simulink model "deltino"  (R2021b)
settings: Solver=VariableStepAuto  StartTime=0.0  StopTime=inf  FixedStep=0.0001  RelTol=1e-3
values from neighbouring files (symbols this model uses):
  alpha1 = 0    [compute_deltino_dyn_parallel.m]
  alpha2 = 2/3*pi    (= 2.09439510239)    [compute_deltino_dyn_parallel.m]
  alpha3 = 4/3*pi    (= 4.18879020479)    [compute_deltino_dyn_parallel.m]
  H = 0.05    [main.m]
  J_T = [J_1', J_2', J_3', J_4']    [main.m]
  K_d = 10    [main.m]
  K_el = 10000    [main.m]
  K_i = 1    [main.m]
  K_p = 200    [main.m]
  K_v = 10    [main.m]
  mu = 0.8    [main.m]
  ni_0 = zeros(18,1)    [main.m]
  offset1 = [l1/2; l2/2; -h/2]    [compute_deltino_dyn_parallel.m]    (also in main.m = [+l1/2; +l2/2; -h/2])
  offset2 = [l1/2; -l2/2; -h/2]    [compute_deltino_dyn_parallel.m]    (also in main.m = [+l1/2; -l2/2; -h/2])
  offset3 = [-l1/2; -l2/2; -h/2]    [compute_deltino_dyn_parallel.m]    (also in main.m)
  offset4 = [-l1/2; l2/2; -h/2]    [compute_deltino_dyn_parallel.m]    (also in main.m = [-l1/2; +l2/2; -h/2])
  p_leg1_0 = forward_kin(theta_leg1_0)    [main.m]
  p_leg2_0 = forward_kin(theta_leg2_0)    [main.m]
  p_leg3_0 = forward_kin(theta_leg3_0)    [main.m]
  p_leg4_0 = forward_kin(theta_leg4_0)    [main.m]
  points_ccw = [+0.1,  0.00 ... (first row only)    [main.m]
  points_cw = [-0.1,  0.00 ... (first row only)    [main.m]
  q_0 = [base_0; ypr_0; theta_leg1_0; ee_leg1_0; theta_leg2_0; ee_leg2_0;        theta_leg3_0; ee_leg3_0; theta_leg4_0; ee_leg4_0;]    [main.m]
  ratio = 2    [main.m]
  steps = 4+2*ratio    (= 8)    [main.m]
  theta_leg1_0 = [pi/6; pi/6; pi/6]    [main.m]
  theta_leg2_0 = [pi/6; pi/6; pi/6]    [main.m]
  theta_leg3_0 = [pi/6; pi/6; pi/6]    [main.m]
  theta_leg4_0 = [pi/6; pi/6; pi/6]    [main.m]
  ts = T/steps    (= 0.1875)    [main.m]
  ts2 = 3*ts    (= 0.5625)    [main.m]
  vel = 0.2    [main.m]
undefined symbols (not defined in the file or in its folder): l1, l_A, l_B, R, radius0, radius1, radius2, theta, WPs
libraries: simulink x14, dspsigops x12
(part 5 of 10)

== matlab function deltino/TRAJ PLANNING/legs traj generator rotate/leg_generator1/MATLAB Function ==
  data: u1 input; y output; u2 input
function y = OR(u1, u2)

if (u1==0) && (u2==0)
    y = 0;
else 
    y = 1;
end

== matlab function deltino/TRAJ PLANNING/legs traj generator rotate/leg_generator1/swing rotate ==
  data: t input; alpha input; pos output; H parameter; ts2 parameter; l1 parameter; offset1 parameter

function pos = fcn(t, alpha, H, ts2, l1, offset1)

T_BD1 = R_z(-(pi+pi/2+pi/4+alpha))*T_x(sqrt(2)*l1/2);
d_B = T_BD1(1:3,4);
d_B1 = d_B - offset1;

x_0 = 0;
x_1 = d_B1(1) ;
    x1 = x_0;
    x2 = 0;
    x3 = 0;
    x4 = (10*(x_1 - x_0))/ts2^3;
    x5 = -(15*(x_1 - x_0))/ts2^4;
    x6 = (6*(x_1 - x_0))/ts2^5;
x = x1 + x2*t + x3*t^2 + x4*t^3 +x5*t^4 + x6*t^5;

y_0 = 0;
y_1 = d_B1(2);
    y1 = y_0;
    y2 = 0;
    y3 = 0;
    y4 = (10*(y_1 - y_0))/ts2^3;
    y5 = -(15*(y_1 - y_0))/ts2^4;
    y6 = (6*(y_1 - y_0))/ts2^5;
y = y1 + y2*t + y3*t^2 + y4*t^3 + y5*t^4 + y6*t^5;

z = H/2*(1 - cos(2*pi*t/ts2));

pos = [x;y;z];

== matlab function deltino/TRAJ PLANNING/legs traj generator rotate/leg_generator2/MATLAB Function ==
  data: u1 input; y output; u2 input
function y = OR(u1, u2)

if (u1==0) && (u2==0)
    y = 0;
else 
    y = 1;
end

== matlab function deltino/TRAJ PLANNING/legs traj generator rotate/leg_generator2/swing rotate ==
  data: t input; alpha input; pos output; H parameter; ts2 parameter; l1 parameter; offset2 parameter

function pos = fcn(t, alpha, H, ts2, l1, offset2)

T_BD2 = R_z(-(pi/4+alpha))*T_x(sqrt(2)*l1/2);
d_B = T_BD2(1:3,4);
d_B2 = d_B - offset2;

x_0 = 0;
x_1 = d_B2(1) ;
    x1 = x_0;
    x2 = 0;
    x3 = 0;
    x4 = (10*(x_1 - x_0))/ts2^3;
    x5 = -(15*(x_1 - x_0))/ts2^4;
    x6 = (6*(x_1 - x_0))/ts2^5;
x = x1 + x2*t + x3*t^2 + x4*t^3 +x5*t^4 + x6*t^5;

y_0 = 0;
y_1 = d_B2(2);
    y1 = y_0;
    y2 = 0;
    y3 = 0;
    y4 = (10*(y_1 - y_0))/ts2^3;
    y5 = -(15*(y_1 - y_0))/ts2^4;
    y6 = (6*(y_1 - y_0))/ts2^5;
y = y1 + y2*t + y3*t^2 + y4*t^3 + y5*t^4 + y6*t^5;

z = H/2*(1 - cos(2*pi*t/ts2));

pos = [x;y;z];

== matlab function deltino/TRAJ PLANNING/ Encoder ==
  data: u1 input; ctrl input; u2 input; y1 output; y2 output; y3 output; y4 output; p_leg2_0 parameter; p_leg1_0 parameter; p_leg3_0 parameter; p_leg4_0 parameter
function [y1, y2, y3, y4] = encoder(u1, ctrl, u2, p_leg2_0, p_leg1_0, p_leg3_0, p_leg4_0)
    y1 = p_leg1_0;
    y2 = p_leg2_0;
    y3 = p_leg3_0;
    y4 = p_leg4_0;
    
    if ctrl == 1 % forth
        y1 = Rz(0)*u1(1:3);
        y2 = Rz(0)*u1(4:6);
        y3 = Rz(0)*u1(7:9);
        y4 = Rz(0)*u1(10:12);
    elseif ctrl == 3 % back
        y1 = Rz(pi)*u1(1:3);
        y2 = Rz(pi)*u1(4:6);
        y3 = Rz(pi)*u1(7:9);
        y4 = Rz(pi)*u1(10:12);
    elseif ctrl == 2 % right
        y1 = Rz(-pi/2)*u1(1:3);
        y2 = Rz(-pi/2)*u1(4:6);
        y3 = Rz(-pi/2)*u1(7:9);
        y4 = Rz(-pi/2)*u1(10:12);
	elseif ctrl == 4 % left
        y1 = Rz(pi/2)*u1(1:3);
        y2 = Rz(pi/2)*u1(4:6);
        y3 = Rz(pi/2)*u1(7:9);
        y4 = Rz(pi/2)*u1(10:12);
    elseif (ctrl == 5) || (ctrl==6)
        y1 = u2(1:3);
        y2 = u2(4:6);
        y3 = u2(7:9);
        y4 = u2(10:12);
    end

== matlab function deltino/TRAJ PLANNING/MATLAB Function ==
  data: mode input; alpha input; real_alpha output
function real_alpha = fcn(mode, alpha)

if mode == 5
    real_alpha = alpha;
else 
    real_alpha = -alpha;
end

== matlab function deltino/TRAJ PLANNING/legs traj generator rotate/leg_generator3/MATLAB Function ==
  data: u1 input; y output; u2 input
function y = OR(u1, u2)

if (u1==0) && (u2==0)
    y = 0;
else 
    y = 1;
end

== matlab function deltino/TRAJ PLANNING/legs traj generator rotate/leg_generator3/swing rotate ==
  data: t input; alpha input; pos output; H parameter; ts2 parameter; l1 parameter; offset3 parameter

function pos = fcn(t, alpha, H, ts2, l1, offset3)

T_BD3 = R_z(-(pi/2+pi/4+alpha))*T_x(sqrt(2)*l1/2);
d_B = T_BD3(1:3,4);
d_B3 = d_B - offset3;

x_0 = 0;
x_1 = d_B3(1) ;
    x1 = x_0;
    x2 = 0;
    x3 = 0;
    x4 = (10*(x_1 - x_0))/ts2^3;
    x5 = -(15*(x_1 - x_0))/ts2^4;
    x6 = (6*(x_1 - x_0))/ts2^5;
x = x1 + x2*t + x3*t^2 + x4*t^3 +x5*t^4 + x6*t^5;

y_0 = 0;
y_1 = d_B3(2);
    y1 = y_0;
    y2 = 0;
    y3 = 0;
    y4 = (10*(y_1 - y_0))/ts2^3;
    y5 = -(15*(y_1 - y_0))/ts2^4;
    y6 = (6*(y_1 - y_0))/ts2^5;
y = y1 + y2*t + y3*t^2 + y4*t^3 + y5*t^4 + y6*t^5;

z = H/2*(1 - cos(2*pi*t/ts2));

pos = [x;y;z];

== matlab function deltino/TRAJ PLANNING/legs traj generator rotate/leg_generator4/MATLAB Function ==
  data: u1 input; y output; u2 input
function y = OR(u1, u2)

if (u1==0) && (u2==0)
    y = 0;
else 
    y = 1;
end

== matlab function deltino/TRAJ PLANNING/legs traj generator rotate/leg_generator4/swing rotate ==
  data: t input; alpha input; pos output; H parameter; ts2 parameter; l1 parameter; offset4 parameter

function pos = fcn(t, alpha, H, ts2, l1, offset4)

T_BD4 = R_z(-(pi+pi/4+alpha))*T_x(sqrt(2)*l1/2);
d_B = T_BD4(1:3,4);
d_B4 = d_B - offset4;

x_0 = 0;
x_1 = d_B4(1) ;
    x1 = x_0;
    x2 = 0;
    x3 = 0;
    x4 = (10*(x_1 - x_0))/ts2^3;
    x5 = -(15*(x_1 - x_0))/ts2^4;
    x6 = (6*(x_1 - x_0))/ts2^5;
x = x1 + x2*t + x3*t^2 + x4*t^3 +x5*t^4 + x6*t^5;

y_0 = 0;
y_1 = d_B4(2);
    y1 = y_0;
    y2 = 0;
    y3 = 0;
    y4 = (10*(y_1 - y_0))/ts2^3;
    y5 = -(15*(y_1 - y_0))/ts2^4;
    y6 = (6*(y_1 - y_0))/ts2^5;
y = y1 + y2*t + y3*t^2 + y4*t^3 + y5*t^4 + y6*t^5;

z = H/2*(1 - cos(2*pi*t/ts2));

pos = [x;y;z];

== matlab function deltino/TRAJ PLANNING/legs traj generator rotate/leg_generator1/swing rotate back ==
  data: t input; alpha input; pos output; ts2 parameter; l1 parameter; offset1 parameter

function pos = fcn(t, alpha, ts2, l1, offset1)

T_BD1 = R_z(-(pi+pi/2+pi/4+alpha))*T_x(sqrt(2)*l1/2);
d_B = T_BD1(1:3,4);
d_B1 = d_B - offset1;

x_0 = d_B1(1);
x_1 = 0;
    x1 = x_0;
    x2 = 0;
    x3 = 0;
    x4 = (10*(x_1 - x_0))/ts2^3;
    x5 = -(15*(x_1 - x_0))/ts2^4;
    x6 = (6*(x_1 - x_0))/ts2^5;
x = x1 + x2*t + x3*t^2 + x4*t^3 +x5*t^4 + x6*t^5;

y_0 = d_B1(2);
y_1 = 0;
    y1 = y_0;
    y2 = 0;
    y3 = 0;
    y4 = (10*(y_1 - y_0))/ts2^3;
    y5 = -(15*(y_1 - y_0))/ts2^4;
    y6 = (6*(y_1 - y_0))/ts2^5;
y = y1 + y2*t + y3*t^2 + y4*t^3 + y5*t^4 + y6*t^5;

pos = [x;y;0];

== matlab function deltino/TRAJ PLANNING/legs traj generator rotate/leg_generator2/swing rotate back ==
  data: t input; alpha input; pos output; ts2 parameter; l1 parameter; offset2 parameter

function pos = fcn(t, alpha, ts2, l1, offset2)

T_BD2 = R_z(-(pi/4+alpha))*T_x(sqrt(2)*l1/2);
d_B = T_BD2(1:3,4);
d_B2 = d_B - offset2;

x_0 = d_B2(1);
x_1 = 0;
    x1 = x_0;
    x2 = 0;
    x3 = 0;
    x4 = (10*(x_1 - x_0))/ts2^3;
    x5 = -(15*(x_1 - x_0))/ts2^4;
    x6 = (6*(x_1 - x_0))/ts2^5;
x = x1 + x2*t + x3*t^2 + x4*t^3 +x5*t^4 + x6*t^5;

y_0 = d_B2(2);
y_1 = 0;
    y1 = y_0;
    y2 = 0;
    y3 = 0;
    y4 = (10*(y_1 - y_0))/ts2^3;
    y5 = -(15*(y_1 - y_0))/ts2^4;
    y6 = (6*(y_1 - y_0))/ts2^5;
y = y1 + y2*t + y3*t^2 + y4*t^3 + y5*t^4 + y6*t^5;

pos = [x;y;0];

== matlab function deltino/TRAJ PLANNING/legs traj generator rotate/leg_generator3/swing rotate back ==
  data: t input; alpha input; pos output; ts2 parameter; l1 parameter; offset3 parameter

function pos = fcn(t, alpha, ts2, l1, offset3)

T_BD3 = R_z(-(pi/2+pi/4+alpha))*T_x(sqrt(2)*l1/2);
d_B = T_BD3(1:3,4);
d_B3 = d_B - offset3;

x_0 = d_B3(1);
x_1 = 0;
    x1 = x_0;
    x2 = 0;
    x3 = 0;
    x4 = (10*(x_1 - x_0))/ts2^3;
    x5 = -(15*(x_1 - x_0))/ts2^4;
    x6 = (6*(x_1 - x_0))/ts2^5;
x = x1 + x2*t + x3*t^2 + x4*t^3 +x5*t^4 + x6*t^5;

y_0 = d_B3(2);
y_1 = 0;
    y1 = y_0;
    y2 = 0;
    y3 = 0;
    y4 = (10*(y_1 - y_0))/ts2^3;
    y5 = -(15*(y_1 - y_0))/ts2^4;
    y6 = (6*(y_1 - y_0))/ts2^5;
y = y1 + y2*t + y3*t^2 + y4*t^3 + y5*t^4 + y6*t^5;

pos = [x;y;0];

== matlab function deltino/TRAJ PLANNING/legs traj generator rotate/leg_generator4/swing rotate back ==
  data: t input; alpha input; pos output; ts2 parameter; l1 parameter; offset4 parameter

function pos = fcn(t, alpha, ts2, l1, offset4)

T_BD4 = R_z(-(pi+pi/4+alpha))*T_x(sqrt(2)*l1/2);
d_B = T_BD4(1:3,4);
d_B4 = d_B - offset4;

x_0 = d_B4(1);
x_1 = 0;
    x1 = x_0;
    x2 = 0;
    x3 = 0;
    x4 = (10*(x_1 - x_0))/ts2^3;
    x5 = -(15*(x_1 - x_0))/ts2^4;
    x6 = (6*(x_1 - x_0))/ts2^5;
x = x1 + x2*t + x3*t^2 + x4*t^3 +x5*t^4 + x6*t^5;

y_0 = d_B4(2);
y_1 = 0;
    y1 = y_0;
    y2 = 0;
    y3 = 0;
    y4 = (10*(y_1 - y_0))/ts2^3;
    y5 = -(15*(y_1 - y_0))/ts2^4;
    y6 = (6*(y_1 - y_0))/ts2^5;
y = y1 + y2*t + y3*t^2 + y4*t^3 + y5*t^4 + y6*t^5;

pos = [x;y;0];

== matlab function deltino/WAYPOINTS GENERATOR/MATLAB Function ==
  data: all_WPs input; old_reached input; current_WP output size=[1,2]; reached input; old_last input; new_last output size=1
function [current_WP, new_last]  = fcn(all_WPs, old_reached, reached, old_last)

dim = size(all_WPs);

if old_last < dim(1)
	if reached == 1 && old_reached == 0
		new_last = old_last + 1;
		current_WP = all_WPs(new_last,:);
	else
		new_last = old_last;
		current_WP = all_WPs(new_last,:);
	end
else
	current_WP = all_WPs(old_last,:);
	new_last = old_last;
end

== matlab function deltino/TRAJ PLANNING/legs traj generator rotate/rotate_CW ==
  data: shift output; leg input; t input; points_cw parameter; ts2 parameter
function shift = shift_CoM(leg, t, points_cw, ts2)

X1 = points_cw(1,1);
Y1 = points_cw(1,2);
X2 = points_cw(2,1);
Y2 = points_cw(2,2);
X3 = points_cw(3,1);
Y3 = points_cw(3,2);


shift = [0;0;0];

switch leg
	case 0.5 
		x_0 = 0;
		x_1 = X1;
		x1 = x_0;
		x2 = 0;
		x3 = 0;
		x4 = (10*(x_1 - x_0))/ts2^3;
		x5 = -(15*(x_1 - x_0))/ts2^4;
		x6 = (6*(x_1 - x_0))/ts2^5;
		shiftx = x1 + x2*t + x3*t^2 + x4*t^3 +x5*t^4 + x6*t^5;
	
		y_0 = 0;
		y_1 = Y1;
		y1 = y_0;
		y2 = 0;
		y3 = 0;
		y4 = (10*(y_1 - y_0))/ts2^3;
		y5 = -(15*(y_1 - y_0))/ts2^4;
		y6 = (6*(y_1 - y_0))/ts2^5;
		shifty = y1 + y2*t + y3*t^2 + y4*t^3 + y5*t^4 + y6*t^5;

		shift = [shiftx; shifty; 0];
	case 1 
		shift = [X1; Y1; 0];
	case 2 
		shift = [X1; Y1; 0];
	case 2.5
		x_0 = X1;
		x_1 = X2;
		x1 = x_0;
		x2 = 0;
		x3 = 0;
		x4 = (10*(x_1 - x_0))/ts2^3;
		x5 = -(15*(x_1 - x_0))/ts2^4;
		x6 = (6*(x_1 - x_0))/ts2^5;
		shiftx = x1 + x2*(t-3*ts2) + x3*(t-3*ts2)^2 + x4*(t-3*ts2)^3 +x5*(t-3*ts2)^4 + x6*(t-3*ts2)^5;
	
		y_0 = Y1;
		y_1 = Y2;
		y1 = y_0;
		y2 = 0;
		y3 = 0;
		y4 = (10*(y_1 - y_0))/ts2^3;
		y5 = -(15*(y_1 - y_0))/ts2^4;
		y6 = (6*(y_1 - y_0))/ts2^5;
		shifty = y1 + y2*(t-3*ts2) + y3*(t-3*ts2)^2 + y4*(t-3*ts2)^3 + y5*(t-3*ts2)^4 + y6*(t-3*ts2)^5;
		shift = [shiftx; shifty; 0];
	case 3
		shift = [X2; Y2; 0];
	case 4 
		shift = [X2; Y2; 0];
	case 5
		x_0 = X2;
		x_1 = X3;
		x1 = x_0;
		x2 = 0;
		x3 = 0;
		x4 = (10*(x_1 - x_0))/ts2^3;
		x5 = -(15*(x_1 - x_0))/ts2^4;
		x6 = (6*(x_1 - x_0))/ts2^5;
		shiftx = x1 + x2*(t-6*ts2) + x3*(t-6*ts2)^2 + x4*(t-6*ts2)^3 +x5*(t-6*ts2)^4 + x6*(t-6*ts2)^5;
	
		y_0 = Y2;
		y_1 = Y3;
		y1 = y_0;
		y2 = 0;
		y3 = 0;
		y4 = (10*(y_1 - y_0))/ts2^3;
		y5 = -(15*(y_1 - y_0))/ts2^4;
		y6 = (6*(y_1 - y_0))/ts2^5;
		shifty = y1 + y2*(t-6*ts2) + y3*(t-6*ts2)^2 + y4*(t-6*ts2)^3 + y5*(t-6*ts2)^4 + y6*(t-6*ts2)^5;
		shift = [shiftx; shifty; 0];
end

% 
% switch leg
% 	case 0.5 
% 		shiftx = X1 * t/ts2;
% 		shifty = Y1 * t/ts2;
% 		shift = [shiftx; shifty; 0];
% 	case 1 
% 		shift = [X1; Y1; 0];
% 	case 2 
% 		shift = [X1; Y1; 0];
% 	case 2.5
% 		shiftx = X2 * (t-3*ts2)/ts2 + X1 * (1-(t-3*ts2)/ts2);
% 		shifty = Y2 * (t-3*ts2)/ts2 + Y1 * (1-(t-3*ts2)/ts2);
% 		shift = [shiftx; shifty; 0];
% 	case 3
% 		shift = [X2; Y2; 0];
% 	case 4 
% 		shift = [X2; Y2; 0];
% 	case 5
% 		shiftx = X3 * (t-6*ts2)/ts2 + X2 * (1-(t-6*ts2)/ts2);
% 		shifty = Y3 * (t-6*ts2)/ts2 + Y2 * (1-(t-6*ts2)/ts2);
% 		shift = [shiftx; shifty; 0];
% end

== matlab function deltino/INVERVSE KINEMATICS/Pos_to_Theta ==
  data: pos_Bi input; alpha1 parameter; alpha2 parameter; alpha3 parameter; R parameter; l_A parameter; l_B parameter; theta output; theta_old output; theta_old input
function [theta, theta_old] = inverse_kin(pos_Bi, alpha1, alpha2, alpha3, R, l_A, l_B, theta_old)

    theta = zeros(12,1);

    for idx = 1:4

        % Foot coordinates in frame {B_i}
        p = pos_Bi(1+(idx-1)*3:idx*3);

        % Equations of trilateration to be solved
        F = @(th) [norm(p - Rz(alpha1) * [R+l_A*cos(th(1)); 0; -l_A*sin(th(1))])^2 - l_B^2;
                   norm(p - Rz(alpha2) * [R+l_A*cos(th(2)); 0; -l_A*sin(th(2))])^2 - l_B^2;
                   norm(p - Rz(alpha3) * [R+l_A*cos(th(3)); 0; -l_A*sin(th(3))])^2 - l_B^2];
        x0 = theta_old(1+(idx-1)*3:idx*3);
        opt = optimoptions('fsolve', 'Algorithm', 'levenberg-marquardt');

        [res, val] = fsolve(F, x0, opt);
        theta(1+(idx-1)*3:idx*3) = res;
    end 
    
    theta_old  = theta;
end

== matlab function deltino/CONTACT FORCES/Contact Forces Leg1/Contact Forces ==
  data: p_ee input; f output; v_ee input; contact input; p0 input; contact output; p0 output; K_el parameter; K_v parameter; mu parameter
function [f, contact, p0] = compute_contact_forces(p_ee, v_ee, contact, p0, K_el, K_v, mu)
    f = zeros(3,1);

    if(p_ee(3) < 0)

        % Normal Force
        f_e = -K_el * p_ee(3);
        if(v_ee(3) < 0)
            f_v = f_e * K_v * (-v_ee(3));
        else
            f_v = 0;
        end
        f(3) = f_e + f_v;

        % Tangential Force
        if(contact == 0) % we must initialize x0
            contact = 1;
            p0 = p_ee(1:2);
            f(1:2) = K_el * (p0 - p_ee(1:2)); % == 0 !! 
        else 
            % tangential force computation
            f(1:2) = K_el * (p0 - p_ee(1:2));

            % update of p0_x  
            if(f(1) > mu * f(3))
                p0(1) = (mu * f(3))/K_el + p_ee(1);
                f(1) = mu * f(3);
            elseif(-f(1) > mu * f(3))
                p0(1) = -(mu * f(3))/K_el + p_ee(1);
                f(1) = - mu * f(3);
            end
            
            % update of p0_y
            if(f(2) > mu * f(3))
                p0(2) = (mu * f(3))/K_el + p_ee(2);
                f(2) = mu * f(3);
            elseif(-f(2) > mu * f(3))
                p0(2) = -(mu * f(3))/K_el + p_ee(2);
              f(2) = -mu * f(3);
            end    
        end
     
    else % reset of contact tracking
        contact = 0;
    end

    %f(1) = 0;
    %f(2) = 0;


end

== matlab function deltino/MATLAB Function1 ==
  data: q input; theta output
function theta = select_theta(q)

theta = [q(7:9); q(13:15); q(19:21); q(25:27)];

end

== matlab function deltino/GUIDANCE SYSTEM/MATLAB Function ==
  data: reached output; mode output; velocity output; wp input; alpha output; q input; doing input; radius0 parameter; vel parameter; old_vel input; old_alpha input; radius1 parameter; radius2 parameter; theta parameter
function [reached, mode, velocity, alpha] = ...
	fcn(wp, q, doing, radius0, vel, old_vel, old_alpha, radius1, radius2, theta)

mode = 0;
alpha = old_alpha;
velocity = old_vel; 
reached = 0;

% DO SOMETHING ONLY IF PREVIOUS ACTION IS FINISHED
if doing == 0 

% 1) Check whether WP is reached
x = wp(1) - q(1);
y = wp(2) - q(2);
dist = sqrt(x^2+y^2);
if dist < radius0 
	reached = 1;
else
	theta = theta/180*pi;

	vel1 = vel/2;
	vel2 = vel/4;
	
	% 2) Check for heading
	robot_yaw = q(4);
	heading_des_spatial = atan2(y,x);
	heading_des_robot = heading_des_spatial-robot_yaw;
	heading_des = wrapToPi(heading_des_robot);
	if (-pi/4 < heading_des) && (heading_des <= pi/4)
    	head = 1; % front
    	heading_des = heading_des+0;
	elseif  (pi/4 < heading_des) && (heading_des <= 3/4*pi)
    	head = 4; % left
    	heading_des = heading_des-pi/2;
	elseif (3/4*pi < heading_des)
    	head = 3; % back
    	heading_des = heading_des-pi;
	elseif (heading_des <= -3/4*pi)
    	head = 3; % back
    	heading_des = heading_des+pi; 
	elseif (-3/4*pi < heading_des) && (heading_des <= -pi/4)
    	head = 2; % right
    	heading_des = heading_des+pi/2;
    else
        head = 9;
	end
	
    miss_distance = abs(dist*sin(heading_des));
    angle_error = abs(heading_des);
	if (angle_error > theta) && (miss_distance > radius0)
		adjust = 1;
	else
		adjust = 0;
	end

	if adjust == 0
    	% 3.1) Adjust velocity
    	mode = head;
		if dist < radius2 
        	velocity = vel2;
    	elseif dist < radius1
        	velocity = vel1;
    	else 
        	velocity = vel;
		end
	else
    	% 3.2) Adjust heading
		if heading_des > 0 % rotate counterclockwise
			if abs(heading_des) <= pi/8 % do just one rotation
				mode = 6;
				alpha = abs(heading_des);
			else %do two rotations
				mode = 6;
				alpha = abs(heading_des)/2;
			end
		else % rotate clockwise
			if abs(heading_des) <= pi/8 % do just one rotation
				mode = 5;
				alpha = abs(heading_des);
			else %do two rotations
				mode = 5;
				alpha = abs(heading_des)/2;
			end
		end
		alpha = alpha + 0.1*alpha;
	end

end

end

== matlab function deltino/TRAJ PLANNING/legs traj generator rotate/rotate CCW ==
  data: shift output; leg input; t input; points_ccw parameter; ts2 parameter
function shift  = shift_CoM(leg, t, points_ccw, ts2)

X1 = points_ccw(1,1);
Y1 = points_ccw(1,2);
X2 = points_ccw(2,1);
Y2 = points_ccw(2,2);
X3 = points_ccw(3,1);
Y3 = points_ccw(3,2);

shift = [0;0;0];

switch leg
	case 4.5 
		x_0 = 0;
		x_1 = X1;
		x1 = x_0;
		x2 = 0;
		x3 = 0;
		x4 = (10*(x_1 - x_0))/ts2^3;
		x5 = -(15*(x_1 - x_0))/ts2^4;
		x6 = (6*(x_1 - x_0))/ts2^5;
		shiftx = x1 + x2*t + x3*t^2 + x4*t^3 +x5*t^4 + x6*t^5;
	
		y_0 = 0;
		y_1 = Y1;
		y1 = y_0;
		y2 = 0;
		y3 = 0;
		y4 = (10*(y_1 - y_0))/ts2^3;
		y5 = -(15*(y_1 - y_0))/ts2^4;
		y6 = (6*(y_1 - y_0))/ts2^5;
		shifty = y1 + y2*t + y3*t^2 + y4*t^3 + y5*t^4 + y6*t^5;

		shift = [shiftx; shifty; 0];
	case 4 
		shift = [X1; Y1; 0];
	case 3 
		shift = [X1; Y1; 0];
	case 2.5
		x_0 = X1;
		x_1 = X2;
		x1 = x_0;
		x2 = 0;
		x3 = 0;
		x4 = (10*(x_1 - x_0))/ts2^3;
		x5 = -(15*(x_1 - x_0))/ts2^4;
		x6 = (6*(x_1 - x_0))/ts2^5;
		shiftx = x1 + x2*(t-3*ts2) + x3*(t-3*ts2)^2 + x4*(t-3*ts2)^3 +x5*(t-3*ts2)^4 + x6*(t-3*ts2)^5;
	
		y_0 = Y1;
		y_1 = Y2;
		y1 = y_0;
		y2 = 0;
		y3 = 0;
		y4 = (10*(y_1 - y_0))/ts2^3;
		y5 = -(15*(y_1 - y_0))/ts2^4;
		y6 = (6*(y_1 - y_0))/ts2^5;
		shifty = y1 + y2*(t-3*ts2) + y3*(t-3*ts2)^2 + y4*(t-3*ts2)^3 + y5*(t-3*ts2)^4 + y6*(t-3*ts2)^5;
		shift = [shiftx; shifty; 0];
	case 2
		shift = [X2; Y2; 0];
	case 1 
		shift = [X2; Y2; 0];
	case 5
		x_0 = X2;
		x_1 = X3;
		x1 = x_0;
		x2 = 0;
		x3 = 0;
		x4 = (10*(x_1 - x_0))/ts2^3;
		x5 = -(15*(x_1 - x_0))/ts2^4;
		x6 = (6*(x_1 - x_0))/ts2^5;
		shiftx = x1 + x2*(t-6*ts2) + x3*(t-6*ts2)^2 + x4*(t-6*ts2)^3 +x5*(t-6*ts2)^4 + x6*(t-6*ts2)^5;
	
		y_0 = Y2;
		y_1 = Y3;
		y1 = y_0;
		y2 = 0;
		y3 = 0;
		y4 = (10*(y_1 - y_0))/ts2^3;
		y5 = -(15*(y_1 - y_0))/ts2^4;
		y6 = (6*(y_1 - y_0))/ts2^5;
		shifty = y1 + y2*(t-6*ts2) + y3*(t-6*ts2)^2 + y4*(t-6*ts2)^3 + y5*(t-6*ts2)^4 + y6*(t-6*ts2)^5;
		shift = [shiftx; shifty; 0];
end

== matlab function deltino/CONTACT FORCES/Contact Forces Leg2/Contact Forces ==
  data: p_ee input; f output; v_ee input; contact input; p0 input; contact output; p0 output; K_el parameter; K_v parameter; mu parameter
function [f, contact, p0] = compute_contact_forces(p_ee, v_ee, contact, p0, K_el, K_v, mu)
    f = zeros(3,1);

    if(p_ee(3) < 0)

        % Normal Force
        f_e = -K_el * p_ee(3);
        if(v_ee(3) < 0)
            f_v = f_e * K_v * (-v_ee(3));
        else
            f_v = 0;
        end
        f(3) = f_e + f_v;

        % Tangential Force
        if(contact == 0) % we must initialize x0
            contact = 1;
            p0 = p_ee(1:2);
            f(1:2) = K_el * (p0 - p_ee(1:2)); % == 0 !! 
        else 
            % tangential force computation
            f(1:2) = K_el * (p0 - p_ee(1:2));

            % update of p0_x  
            if(f(1) > mu * f(3))
                p0(1) = (mu * f(3))/K_el + p_ee(1);
                f(1) = mu * f(3);
            elseif(-f(1) > mu * f(3))
                p0(1) = -(mu * f(3))/K_el + p_ee(1);
                f(1) = - mu * f(3);
            end
            
            % update of p0_y
            if(f(2) > mu * f(3))
                p0(2) = (mu * f(3))/K_el + p_ee(2);
                f(2) = mu * f(3);
            elseif(-f(2) > mu * f(3))
                p0(2) = -(mu * f(3))/K_el + p_ee(2);
              f(2) = -mu * f(3);
            end    
        end
     
    else % reset of contact tracking
        contact = 0;
    end
    
    %f(1) = 0;
    %f(2) = 0;


end

== matlab function deltino/TRAJ PLANNING/MATLAB Function1 ==
  data: u input; y output
function y = fcn(u)
if u==1
	y = 0;
else
	y = 1;
end

== matlab function deltino/TRAJ PLANNING/legs traj generator move/leg_generator1/MATLAB Function ==
  data: u input; y output
function y = fcn(u)

y = u(1);

== stateflow chart deltino/TRAJ PLANNING/Chart2 ==
  state MoveRobot
    du: reset = 0;
    en: reset1 = 1;
    en: reset2 = 1;
    en: reset3 = 1;
    en: reset4 = 1;
    state MoveForth1
      state MoveRobot2
        en: leg=2;
        en: reset3 = 1;
      state MoveRobot1
        en: leg=0;
      state MoveRobot5
        en: leg=3;
        en: reset1 = 0;
        en:reset2 = 0;
        en:reset3 = 0;
        en:reset4 = 0;
      state MoveRobot7
        en: leg=0;
        en: reset1 = 1;
      state MoveRobot6
        entry: leg=0;
        en: reset2 = 1;
      state MoveRobot3
        entry: leg=4;
      state MoveRobot4
        entry: leg = 1;
        en: reset4 = 1;
      (default) -> MoveRobot.MoveForth1.MoveRobot1
      MoveRobot.MoveForth1.MoveRobot5 -> MoveRobot.MoveForth1.MoveRobot2 : [after(ts,sec)]
      MoveRobot.MoveForth1.MoveRobot1 -> MoveRobot.MoveForth1.MoveRobot5 : [after(0.5*ratio*ts, sec)]
      MoveRobot.MoveForth1.MoveRobot2 -> MoveRobot.MoveForth1.MoveRobot6 : [after(ts,sec)]
      MoveRobot.MoveForth1.MoveRobot4 -> MoveRobot.MoveForth1.MoveRobot7 : [after(ts,sec)]
      MoveRobot.MoveForth1.MoveRobot6 -> MoveRobot.MoveForth1.MoveRobot3 : [after(ratio*ts, sec)]
      MoveRobot.MoveForth1.MoveRobot3 -> MoveRobot.MoveForth1.MoveRobot4 : [after(ts,sec)]
    state MoveRight1
      state MoveRobot2
        en: leg=3;
        en: reset4 = 1;
      state MoveRobot1
        entry: leg=0;
      state MoveRobot5
        entry: leg=4;
        en:reset1 = 0;
        en:reset2 = 0;
        en:reset3 = 0;
        en:reset4 = 0;
      state MoveRobot7
        entry: leg=0;
        en: reset2 = 1;
      state MoveRobot6
        entry: leg=0;
        en: reset3 = 1;
      state MoveRobot3
        entry: leg=1;
      state MoveRobot4
        entry: leg = 2;
        en: reset1 = 1;
      (default) -> MoveRobot.MoveRight1.MoveRobot1
      MoveRobot.MoveRight1.MoveRobot5 -> MoveRobot.MoveRight1.MoveRobot2 : [after(ts,sec)]
      MoveRobot.MoveRight1.MoveRobot1 -> MoveRobot.MoveRight1.MoveRobot5 : [after(0.5*ratio*ts, sec)]
      MoveRobot.MoveRight1.MoveRobot2 -> MoveRobot.MoveRight1.MoveRobot6 : [after(ts,sec)]
      MoveRobot.MoveRight1.MoveRobot4 -> MoveRobot.MoveRight1.MoveRobot7 : [after(ts,sec)]
      MoveRobot.MoveRight1.MoveRobot6 -> MoveRobot.MoveRight1.MoveRobot3 : [after(ratio*ts, sec)]
      MoveRobot.MoveRight1.MoveRobot3 -> MoveRobot.MoveRight1.MoveRobot4 : [after(ts,sec)]
    state MoveForth2
      state MoveRobot2
        en: leg=1;
        en: reset4 = 1;
      state MoveRobot1
        en: leg=0;
      state MoveRobot5
        en: leg=4;
        en:reset1 = 0;
        en:reset2 = 0;
        en:reset3 = 0;
        en:reset4 = 0;
      state MoveRobot6
        en: leg=0;
        en: reset1 = 1;
      state MoveRobot7
        entry: leg=0;
        en:reset2 = 1;
      state MoveRobot4
        entry: leg = 2;
        en: reset3 = 1;
      state MoveRobot3
        en: leg=3;
      (default) -> MoveRobot.MoveForth2.MoveRobot1
      MoveRobot.MoveForth2.MoveRobot5 -> MoveRobot.MoveForth2.MoveRobot2 : [after(ts,sec)]
      MoveRobot.MoveForth2.MoveRobot1 -> MoveRobot.MoveForth2.MoveRobot5 : [after(0.5*ratio*ts, sec)]
      MoveRobot.MoveForth2.MoveRobot2 -> MoveRobot.MoveForth2.MoveRobot6 : [after(ts,sec)]
      MoveRobot.MoveForth2.MoveRobot6 -> MoveRobot.MoveForth2.MoveRobot3 : [after(ratio*ts, sec)]
      MoveRobot.MoveForth2.MoveRobot4 -> MoveRobot.MoveForth2.MoveRobot7 : [after(ts,sec)]
      MoveRobot.MoveForth2.MoveRobot3 -> MoveRobot.MoveForth2.MoveRobot4 : [after(ts,sec)]
    state MoveRight2
      state MoveRobot2
        en: leg=2;
        en: reset1 = 1;
      state MoveRobot1
        entry: leg=0;
      state MoveRobot5
        entry: leg=1;
        en:reset1 = 0;
        en:reset2 = 0;
        en:reset3 = 0;
        en:reset4 = 0;
      state MoveRobot6
        entry: leg=0;
        en: reset2 = 1;
      state MoveRobot7
        entry: leg=0;
        en: reset3 = 1;
      state MoveRobot4
        entry: leg = 3;
        en: reset4 = 1;
      state MoveRobot3
        entry: leg=4;
      (default) -> MoveRobot.MoveRight2.MoveRobot1
      MoveRobot.MoveRight2.MoveRobot5 -> MoveRobot.MoveRight2.MoveRobot2 : [after(ts,sec)]
      MoveRobot.MoveRight2.MoveRobot1 -> MoveRobot.MoveRight2.MoveRobot5 : [after(0.5*ratio*ts, sec)]
      MoveRobot.MoveRight2.MoveRobot2 -> MoveRobot.MoveRight2.MoveRobot6 : [after(ts,sec)]
      MoveRobot.MoveRight2.MoveRobot6 -> MoveRobot.MoveRight2.MoveRobot3 : [after(ratio*ts, sec)]
      MoveRobot.MoveRight2.MoveRobot4 -> MoveRobot.MoveRight2.MoveRobot7 : [after(ts,sec)]
      MoveRobot.MoveRight2.MoveRobot3 -> MoveRobot.MoveRight2.MoveRobot4 : [after(ts,sec)]
    state MoveLeft1
      state MoveRobot2
        en: leg=1;
        en:reset2 = 1;
      state MoveRobot1
        entry: leg=0;
      state MoveRobot5
        entry: leg=2;
        en:reset1 = 0;
        en:reset2 = 0;
        en:reset3 = 0;
        en:reset4 = 0;
      state MoveRobot7
        entry: leg=0;
        en: reset4 = 1;
      state MoveRobot6
        entry: leg=0;
        en: reset1 = 1;
      state MoveRobot3
        entry: leg=3;
      state MoveRobot4
        entry: leg = 4;
        en: reset3 = 1;
      (default) -> MoveRobot.MoveLeft1.MoveRobot1
      MoveRobot.MoveLeft1.MoveRobot5 -> MoveRobot.MoveLeft1.MoveRobot2 : [after(ts,sec)]
      MoveRobot.MoveLeft1.MoveRobot1 -> MoveRobot.MoveLeft1.MoveRobot5 : [after(0.5*ratio*ts, sec)]
      MoveRobot.MoveLeft1.MoveRobot2 -> MoveRobot.MoveLeft1.MoveRobot6 : [after(ts,sec)]
      MoveRobot.MoveLeft1.MoveRobot4 -> MoveRobot.MoveLeft1.MoveRobot7 : [after(ts,sec)]
      MoveRobot.MoveLeft1.MoveRobot6 -> MoveRobot.MoveLeft1.MoveRobot3 : [after(ratio*ts, sec)]
      MoveRobot.MoveLeft1.MoveRobot3 -> MoveRobot.MoveLeft1.MoveRobot4 : [after(ts,sec)]
    state MoveBack1
      state MoveRobot2
        en: leg=4;
        en: reset1 = 1;
      state MoveRobot1
        entry: leg=0;
      state MoveRobot5
        entry: leg=1;
        en:reset1 = 0;
        en:reset2 = 0;
        en:reset3 = 0;
        en:reset4 = 0;
      state MoveRobot7
        entry: leg=0;
        en: reset3 = 1;
      state MoveRobot6
        entry: leg=0;
        en: reset4 = 1;
      state MoveRobot3
        entry: leg=2;
      state MoveRobot4
        entry: leg = 3;
        en: reset2 = 1;
      (default) -> MoveRobot.MoveBack1.MoveRobot1
      MoveRobot.MoveBack1.MoveRobot5 -> MoveRobot.MoveBack1.MoveRobot2 : [after(ts,sec)]
      MoveRobot.MoveBack1.MoveRobot1 -> MoveRobot.MoveBack1.MoveRobot5 : [after(0.5*ratio*ts, sec)]
      MoveRobot.MoveBack1.MoveRobot2 -> MoveRobot.MoveBack1.MoveRobot6 : [after(ts,sec)]
      MoveRobot.MoveBack1.MoveRobot4 -> MoveRobot.MoveBack1.MoveRobot7 : [after(ts,sec)]
      MoveRobot.MoveBack1.MoveRobot6 -> MoveRobot.MoveBack1.MoveRobot3 : [after(ratio*ts, sec)]
      MoveRobot.MoveBack1.MoveRobot3 -> MoveRobot.MoveBack1.MoveRobot4 : [after(ts,sec)]
    state MoveBack2
      state MoveRobot2
        en: leg=3;
        en: reset2 = 1;
      state MoveRobot1
        entry: leg=0;
      state MoveRobot5
        entry: leg=2;
        en:reset1 = 0;
        en:reset2 = 0;
        en:reset3 = 0;
        en:reset4 = 0;
      state MoveRobot6
        entry: leg=0;
        en: reset3 = 1;
      state MoveRobot7
        entry: leg=0;
        en: reset4 = 1;
      state MoveRobot4
        entry: leg = 4;
        en: reset1 = 1;
      state MoveRobot3
        entry: leg=1;
      (default) -> MoveRobot.MoveBack2.MoveRobot1
      MoveRobot.MoveBack2.MoveRobot5 -> MoveRobot.MoveBack2.MoveRobot2 : [after(ts,sec)]
      MoveRobot.MoveBack2.MoveRobot1 -> MoveRobot.MoveBack2.MoveRobot5 : [after(0.5*ratio*ts, sec)]
      MoveRobot.MoveBack2.MoveRobot2 -> MoveRobot.MoveBack2.MoveRobot6 : [after(ts,sec)]
      MoveRobot.MoveBack2.MoveRobot6 -> MoveRobot.MoveBack2.MoveRobot3 : [after(ratio*ts, sec)]
      MoveRobot.MoveBack2.MoveRobot4 -> MoveRobot.MoveBack2.MoveRobot7 : [after(ts,sec)]
      MoveRobot.MoveBack2.MoveRobot3 -> MoveRobot.MoveBack2.MoveRobot4 : [after(ts,sec)]
    state MoveLeft2
      state MoveRobot2
        en: leg=4;
        en: reset3 = 1;
      state MoveRobot1
        entry: leg=0;
      state MoveRobot5
        entry: leg=3;
        en:reset1 = 0;
        en:reset2 = 0;
        en:reset3 = 0;
        en:reset4 = 0;
      state MoveRobot6
        entry: leg=0;
        en: reset4 = 1;
      state MoveRobot7
        entry: leg=0;
        en: reset1 = 1;
      state MoveRobot4
        entry: leg = 1;
        en: reset2 = 1;
      state MoveRobot3
        entry: leg=2;
      (default) -> MoveRobot.MoveLeft2.MoveRobot1
      MoveRobot.MoveLeft2.MoveRobot5 -> MoveRobot.MoveLeft2.MoveRobot2 : [after(ts,sec)]
      MoveRobot.MoveLeft2.MoveRobot1 -> MoveRobot.MoveLeft2.MoveRobot5 : [after(0.5*ratio*ts, sec)]
      MoveRobot.MoveLeft2.MoveRobot2 -> MoveRobot.MoveLeft2.MoveRobot6 : [after(ts,sec)]
      MoveRobot.MoveLeft2.MoveRobot6 -> MoveRobot.MoveLeft2.MoveRobot3 : [after(ratio*ts, sec)]
      MoveRobot.MoveLeft2.MoveRobot4 -> MoveRobot.MoveLeft2.MoveRobot7 : [after(ts,sec)]
      MoveRobot.MoveLeft2.MoveRobot3 -> MoveRobot.MoveLeft2.MoveRobot4 : [after(ts,sec)]
    (junction 159) -> MoveRight1 [order 1] : [type==0]{type =1;}
    (junction 159) -> MoveRight2 [order 2] : {type = 0;}
    (junction 101) -> MoveForth1 [order 1] : [type==0]
        | {type =1;}
    (junction 101) -> MoveForth2 [order 2] : {type = 0;}
    (junction 338) -> MoveLeft1 [order 1] : [type==0]{type =1;}
    (junction 371) -> MoveBack1 [order 1] : [type==0]{type =1;}
    (junction 338) -> MoveLeft2 [order 2] : {type = 0;}
    (junction 371) -> MoveBack2 [order 2] : {type = 0;}
  state RotateRobot
    du: reset = 0;
    state clockwise
      du: mode = 5;
      state cw1
        leg = 0.5;
      state cw2
        leg = 1;
      state cw3
        leg = 2;
      state cw7
        leg = 5;
      state cw4
        leg = 2.5;
      state cw5
        leg = 3;
      state cw6
        leg = 4;
      cw1 -> cw2 : [after(ts2,sec)]
      cw2 -> cw3 : [after(ts2,sec)]
      (default) -> cw1
      cw3 -> cw4 : [after(ts2,sec)]
      cw6 -> cw7 : [after(ts2,sec)]
      cw4 -> cw5 : [after(ts2,sec)]
      cw5 -> cw6 : [after(ts2,sec)]
    state counterclockwise
      du: mode = 6;
      state ccw1
        leg = 4.5;
      state ccw2
        leg = 4;
      state ccw3
        leg = 3;
      state ccw7
        leg = 5;
      state ccw4
        leg = 2.5;
      state ccw5
        leg = 2;
      state ccw6
        leg = 1;
      ccw1 -> ccw2 : [after(ts2,sec)]
      ccw2 -> ccw3 : [after(ts2,sec)]
      (default) -> ccw1
      ccw3 -> ccw4 : [after(ts2,sec)]
      ccw6 -> ccw7 : [after(ts2,sec)]
      ccw4 -> ccw5 : [after(ts2,sec)]
      ccw5 -> ccw6 : [after(ts2,sec)]
  state Wait
    du: reset=1;
    du:reset1 = 0;
    du: leg = 0;
    du: mode = 0;
  Wait -> (junction 159) [order 2] : [cmd==2]{mode=2;}
  Wait -> (junction 101) [order 3] : [cmd==1]{mode =1;}
  (default) -> Wait
  Wait -> clockwise [order 5] : [cmd==5]
      | {mode=5;leg = 0.5;}
  MoveRobot -> Wait : [time>=steps*ts]
      | {reset=1;mode = 0;
      | reset1 = 0;reset2 = 0;reset3 = 0;reset4 = 0;}
  RotateRobot -> Wait : [after(7*ts2, sec)]
      | {reset=1;}
  Wait -> counterclockwise [order 6] : [cmd==6]
      | {mode=6;leg=4.5;}
  Wait -> (junction 371) [order 4] : [cmd==3]{mode =3;}
  Wait -> (junction 338) [order 1] : [cmd==4]{mode =4;}
  data: time input; cmd input; reset output; leg output; ts parameter; mode output; type local =0; steps parameter; ratio parameter; ts2 parameter; reset1 output; reset2 output; reset3 output; reset4 output

== matlab function deltino/TRAJ PLANNING/legs traj generator move/leg_generator1/shift backward ==
  data: vel input; t input; x_0 input; pos output; ts parameter
function pos = fcn(vel, t, x_0, ts)

x_0 = x_0(1);
if x_0 > 0 
    n = round(x_0 / (ts*vel));
    x_0 = n*ts*vel;
end
x = x_0 - vel*t;
pos = [x;0;0];

== matlab function deltino/TRAJ PLANNING/legs traj generator move/leg_generator1/MATLAB Function1 ==
  data: u input; y output
function y = fcn(u)

y = u(1);

== matlab function deltino/TRAJ PLANNING/legs traj generator move/leg_generator2/MATLAB Function ==
  data: u input; y output
function y = fcn(u)

y = u(1);

== matlab function deltino/CONTACT FORCES/Contact Forces Leg3/Contact Forces ==
  data: p_ee input; f output; v_ee input; contact input; p0 input; contact output; p0 output; K_el parameter; K_v parameter; mu parameter
function [f, contact, p0] = compute_contact_forces(p_ee, v_ee, contact, p0, K_el, K_v, mu)
    f = zeros(3,1);

    if(p_ee(3) < 0)

        % Normal Force
        f_e = -K_el * p_ee(3);
        if(v_ee(3) < 0)
            f_v = f_e * K_v * (-v_ee(3));
        else
            f_v = 0;
        end
        f(3) = f_e + f_v;

        % Tangential Force
        if(contact == 0) % we must initialize x0
            contact = 1;
            p0 = p_ee(1:2);
            f(1:2) = K_el * (p0 - p_ee(1:2)); % == 0 !! 
        else 
            % tangential force computation
            f(1:2) = K_el * (p0 - p_ee(1:2));

            % update of p0_x  
            if(f(1) > mu * f(3))
                p0(1) = (mu * f(3))/K_el + p_ee(1);
                f(1) = mu * f(3);
            elseif(-f(1) > mu * f(3))
                p0(1) = -(mu * f(3))/K_el + p_ee(1);
                f(1) = - mu * f(3);
            end
            
            % update of p0_y
            if(f(2) > mu * f(3))
                p0(2) = (mu * f(3))/K_el + p_ee(2);
                f(2) = mu * f(3);
            elseif(-f(2) > mu * f(3))
                p0(2) = -(mu * f(3))/K_el + p_ee(2);
              f(2) = -mu * f(3);
            end    
        end
     
    else % reset of contact tracking
        contact = 0;
    end
    
    %f(1) = 0;
    %f(2) = 0;


end

== matlab function deltino/CONTACT FORCES/Contact Forces Leg4/Contact Forces ==
  data: p_ee input; f output; v_ee input; contact input; p0 input; contact output; p0 output; K_el parameter; K_v parameter; mu parameter
function [f, contact, p0] = compute_contact_forces(p_ee, v_ee, contact, p0, K_el, K_v, mu)
    f = zeros(3,1);

    if(p_ee(3) < 0)

        % Normal Force
        f_e = -K_el * p_ee(3);
        if(v_ee(3) < 0)
            f_v = f_e * K_v * (-v_ee(3));
        else
            f_v = 0;
        end
        f(3) = f_e + f_v;

        % Tangential Force
        if(contact == 0) % we must initialize x0
            contact = 1;
            p0 = p_ee(1:2);
            f(1:2) = K_el * (p0 - p_ee(1:2)); % == 0 !! 
        else 
            % tangential force computation
            f(1:2) = K_el * (p0 - p_ee(1:2));

            % update of p0_x  
            if(f(1) > mu * f(3))
                p0(1) = (mu * f(3))/K_el + p_ee(1);
                f(1) = mu * f(3);
            elseif(-f(1) > mu * f(3))
                p0(1) = -(mu * f(3))/K_el + p_ee(1);
                f(1) = - mu * f(3);
            end
            
            % update of p0_y
            if(f(2) > mu * f(3))
                p0(2) = (mu * f(3))/K_el + p_ee(2);
                f(2) = mu * f(3);
            elseif(-f(2) > mu * f(3))
                p0(2) = -(mu * f(3))/K_el + p_ee(2);
              f(2) = -mu * f(3);
            end    
        end
     
    else % reset of contact tracking
        contact = 0;
    end
    
    %f(1) = 0;
    %f(2) = 0;


end

== matlab function deltino/CONTACT FORCES/MATLAB Function1 ==
  data: q input; ee_leg1 output; ee_leg2 output; ee_leg3 output; ee_leg4 output
function [ee_leg1, ee_leg2, ee_leg3, ee_leg4] = split(q)

    ee_leg1 = q(10:12);
    ee_leg2 = q(16:18);
    ee_leg3 = q(22:24);
    ee_leg4 = q(28:30);
    
end

== matlab function deltino/TRAJ PLANNING/legs traj generator move/leg_generator1/swing forward ==
  data: x_0 input; t input; pos output; H parameter; steps parameter; vel input; ts parameter

function pos = fcn(x_0, t, H, steps, vel, ts)

x_0 = x_0(1);
x_1 = x_0 + vel*(steps-1)*ts;

    x1 = x_0;
    x2 = -vel;
    x3 = 0;
    x4 = (10*(x_1 - x_0 + ts*vel))/ts^3;
    x5 = -(15*(x_1 - x_0 + ts*vel))/ts^4;
    x6 = (6*(x_1 - x_0 + ts*vel))/ts^5;

x = x1 + x2*t + x3*t^2 + x4*t^3 +x5*t^4 + x6*t^5;
z = H/2*(1 - cos(2*pi*t/ts));

pos = [x;0;z];

== matlab function deltino/DELTINO DYNAMICS /MATLAB Function2 ==
  data: S_dot input; C input; G input; M input; S input; tau input; tau_contact input size=[30;1]; ni_dot output size=[18;1]; ni input
function ni_dot = compute_ni_dot(S_dot, C, G, M, S, tau, tau_contact, ni)

    ni_dot = (S'*M*S)\S'*(tau + tau_contact -(M*S_dot+C*S)*ni-G); 

end

== matlab function deltino/CONTACT FORCES/MATLAB Function3 ==
  data: q_dot input; ee_dot_leg1 output; ee_dot_leg2 output; ee_dot_leg3 output; ee_dot_leg4 output
function [ee_dot_leg1, ee_dot_leg2, ee_dot_leg3, ee_dot_leg4] = split2(q_dot)

    ee_dot_leg1 = q_dot(10:12);
    ee_dot_leg2 = q_dot(16:18);
    ee_dot_leg3 = q_dot(22:24);
    ee_dot_leg4 = q_dot(28:30);
    
end

== matlab function deltino/TRAJ PLANNING/legs traj generator move/leg_generator2/MATLAB Function1 ==
  data: u input; y output
function y = fcn(u)

y = u(1);

== matlab function deltino/TRAJ PLANNING/legs traj generator move/leg_generator2/shift backward ==
  data: vel input; t input; x_0 input; pos output; ts parameter
function pos = fcn(vel, t, x_0, ts)

x_0 = x_0(1);
if x_0 > 0 
    n = round(x_0 / (ts*vel));
    x_0 = n*ts*vel;
end
x = x_0 - vel*t;
pos = [x;0;0];

== matlab function deltino/DELTINO DYNAMICS /assign_tau ==
  data: tau input; tau_f output size=[30;1]
function tau_f = assign_tau(tau)
    tau_f = zeros(30,1);
    tau_f(7:9) = tau(1:3);
    tau_f(13:15) = tau(4:6);
    tau_f(19:21) = tau(7:9);
    tau_f(25:27) = tau(10:12);
end

== matlab function deltino/TRAJ PLANNING/legs traj generator move/leg_generator2/swing forward ==
  data: x_0 input; t input; pos output; H parameter; steps parameter; vel input; ts parameter

function pos = fcn(x_0, t, H, steps, vel, ts)

x_0 = x_0(1);
x_1 = x_0 + vel*(steps-1)*ts;

    x1 = x_0;
    x2 = -vel;
    x3 = 0;
    x4 = (10*(x_1 - x_0 + ts*vel))/ts^3;
    x5 = -(15*(x_1 - x_0 + ts*vel))/ts^4;
    x6 = (6*(x_1 - x_0 + ts*vel))/ts^5;

x = x1 + x2*t + x3*t^2 + x4*t^3 +x5*t^4 + x6*t^5;
z = H/2*(1 - cos(2*pi*t/ts));

pos = [x;0;z];

== matlab function deltino/TRAJ PLANNING/legs traj generator move/leg_generator3/MATLAB Function ==
  data: u input; y output
function y = fcn(u)

y = u(1);

== matlab function deltino/TRAJ PLANNING/legs traj generator move/leg_generator3/MATLAB Function1 ==
  data: u input; y output
function y = fcn(u)

y = u(1);

== matlab function deltino/TRAJ PLANNING/legs traj generator move/leg_generator3/shift backward ==
  data: vel input; t input; x_0 input; pos output; ts parameter
function pos = fcn(vel, t, x_0, ts)

x_0 = x_0(1);
if x_0 > 0 
    n = round(x_0 / (ts*vel));
    x_0 = n*ts*vel;
end
x = x_0 - vel*t;
pos = [x;0;0];

== matlab function deltino/TRAJ PLANNING/legs traj generator move/leg_generator3/swing forward ==
  data: x_0 input; t input; pos output; H parameter; steps parameter; vel input; ts parameter

function pos = fcn(x_0, t, H, steps, vel, ts)

x_0 = x_0(1);
x_1 = x_0 + vel*(steps-1)*ts;

    x1 = x_0;
    x2 = -vel;
    x3 = 0;
    x4 = (10*(x_1 - x_0 + ts*vel))/ts^3;
    x5 = -(15*(x_1 - x_0 + ts*vel))/ts^4;
    x6 = (6*(x_1 - x_0 + ts*vel))/ts^5;

x = x1 + x2*t + x3*t^2 + x4*t^3 +x5*t^4 + x6*t^5;
z = H/2*(1 - cos(2*pi*t/ts));

pos = [x;0;z];

== matlab function deltino/TRAJ PLANNING/legs traj generator move/leg_generator4/MATLAB Function ==
  data: u input; y output
function y = fcn(u)

y = u(1);

== matlab function deltino/TRAJ PLANNING/legs traj generator move/leg_generator4/MATLAB Function1 ==
  data: u input; y output
function y = fcn(u)

y = u(1);

== matlab function deltino/TRAJ PLANNING/legs traj generator move/leg_generator4/shift backward ==
  data: vel input; t input; x_0 input; pos output; ts parameter
function pos = fcn(vel, t, x_0, ts)

x_0 = x_0(1);
if x_0 > 0 
    n = round(x_0 / (ts*vel));
    x_0 = n*ts*vel;
end
x = x_0 - vel*t;
pos = [x;0;0];

== matlab function deltino/TRAJ PLANNING/legs traj generator move/leg_generator4/swing forward ==
  data: x_0 input; t input; pos output; H parameter; steps parameter; vel input; ts parameter

function pos = fcn(x_0, t, H, steps, vel, ts)

x_0 = x_0(1);
x_1 = x_0 + vel*(steps-1)*ts;

    x1 = x_0;
    x2 = -vel;
    x3 = 0;
    x4 = (10*(x_1 - x_0 + ts*vel))/ts^3;
    x5 = -(15*(x_1 - x_0 + ts*vel))/ts^4;
    x6 = (6*(x_1 - x_0 + ts*vel))/ts^5;

x = x1 + x2*t + x3*t^2 + x4*t^3 +x5*t^4 + x6*t^5;
z = H/2*(1 - cos(2*pi*t/ts));

pos = [x;0;z];
